simulink model "simulation"  (R2016b)
settings: Solver=ode45  StartTime=0.0  StopTime=1500  RelTol=1e-3  EnableMultiTasking=on
undefined symbols (not defined in the file or in its folder): model
settings Model: Creator=schauer  LastModifiedBy=schauer
settings DataIOCC: LimitDataPoints=on  SaveFormat=Array
settings OptimizationCC: LifeSpan=inf
settings DebuggingCC: SolverPrmCheckMsg=warning  SFUnexpectedBacktrackingDiag=warning  SFNoUnconditionalDefaultTransitionDiag=warning  SFExecutionAtInitializationDiag=none
settings HardwareCC: ProdBitPerPointer=32  ProdBitPerSizeT=32  ProdBitPerPtrDiffT=32  ProdLargestAtomicFloat=None  ProdIntDivRoundTo=Undefined  ProdEndianess=Unspecified  ProdWordSize=32  ProdHWDeviceType=32-bit Generic
settings ModelReferenceCC: PropagateSignalLabelsOutOfModel=off
settings GRTTargetCC: TargetLangStandard=C89/C90 (ANSI)  GeneratePreprocessorConditionals=Disable all
settings ConfigComp: CovMetricSettings=dw  CovHtmlReporting=on  CovSaveCumulativeToWorkspaceVar=on  CovSaveSingleToWorkspaceVar=on  CovExternalEMLEnable=off  CovSFcnEnable=off

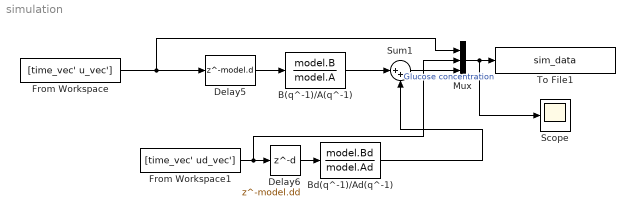
== system simulation ==
  B(q^-1)/A(q^-1) : DiscreteFilter  Numerator=model.B  Denominator=model.A
  Bd(q^-1)/Ad(q^-1) : DiscreteFilter  Numerator=model.Bd  Denominator=model.Ad
  Delay5 : Delay  DelayLength=model.d  InitialCondition=0  SampleTime=model.Ts
  Delay6 : Delay  DelayLength=model.dd  InitialCondition=0  SampleTime=model.Ts
  From Workspace : FromWorkspace  VariableName=[time_vec' u_vec']  SampleTime=0  Interpolate=off  OutputAfterFinalValue=Setting to zero
  From Workspace1 : FromWorkspace  VariableName=[time_vec' ud_vec']  SampleTime=0  Interpolate=off  OutputAfterFinalValue=Setting to zero
  Mux : Mux  Inputs=3
  Scope : Scope
  Sum1 : Sum  Inputs=|++
  To File1 : ToFile  Filename=sim_data  MatrixName=data  SampleTime=model.Ts
  wires:
  From Workspace1/1 -> Delay6/1, Mux/2
  From Workspace/1 -> Mux/1, Delay5/1
  Bd(q^-1)/Ad(q^-1)/1 -> Sum1/2
  B(q^-1)/A(q^-1)/1 -> Sum1/1
  Delay6/1 -> Bd(q^-1)/Ad(q^-1)/1
  Delay5/1 -> B(q^-1)/A(q^-1)/1
  Sum1/1 -> Mux/3  "Glucose concentration"
  Mux/1 -> Scope/1, To File1/1
